simulink model "Test_Encoder_4_to_2"  (Simulink 8.1)
settings: Solver=ode45  StartTime=0.0  StopTime=len  RelTol=1e-3
libraries: commutil2 x2, Encoders_Lib x1
settings Model: Creator=N  LastModifiedBy=uzivatel
settings DataIOCC: LimitDataPoints=off  SignalLoggingSaveFormat=Dataset
settings OptimizationCC: ExpressionDepthLimit=128
settings DebuggingCC: UnderspecifiedInitializationDetection=Simplified  MergeDetectMultiDrivingBlocksExec=error  SolverPrmCheckMsg=none  FcnCallInpInsideContextMsg=EnableAllAsError  FrameProcessingCompatibilityMsg=error  StateNameClashWarn=none
settings HardwareCC: ProdBitPerPointer=64  ProdLargestAtomicFloat=Float  ProdIntDivRoundTo=Zero  ProdEndianess=LittleEndian  ProdHWDeviceType=Intel->x86-64 (Windows64)
settings ModelReferenceCC: PropagateSignalLabelsOutOfModel=on
settings GRTTargetCC: CodeReplacementLibrary=None  CombineOutputUpdateFcns=on  CPPClassGenCompliant=on  GRTInterface=off

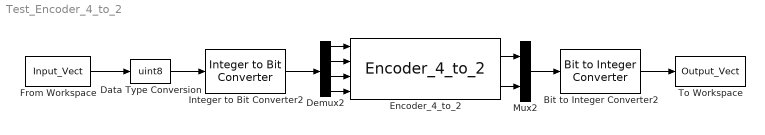
== system Test_Encoder_4_to_2 ==
  Bit to Integer Converter2 : commutil2/Bit to Integer Converter  nbits=2  bitOrder=MSB first  signedOutputValues=Unsigned  outDtype=uint8  outDtypeSigned=Inherit via internal rule
  Data Type Conversion : DataTypeConversion  OutDataTypeStr=uint8
  Demux2 : Demux
  Encoder_4_to_2 : Encoders_Lib/Encoders_Lib/Encoder_4_to_2
  From Workspace : FromWorkspace  VariableName=Input_Vect  SampleTime=1  Interpolate=off  OutputAfterFinalValue=Holding final value
  Integer to Bit Converter2 : commutil2/Integer to Bit Converter  nbits=4  signedInputValues=Unsigned  bitOrder=MSB first  outDtype=boolean
  Mux2 : Mux  Inputs=2
  To Workspace : ToWorkspace  VariableName=Output_Vect  SampleTime=1
  wires:
  Integer to Bit Converter2/1 -> Demux2/1
  Demux2/4 -> Encoder_4_to_2/4
  Demux2/3 -> Encoder_4_to_2/3
  Demux2/2 -> Encoder_4_to_2/2
  Demux2/1 -> Encoder_4_to_2/1
  Mux2/1 -> Bit to Integer Converter2/1
  Bit to Integer Converter2/1 -> To Workspace/1
  Encoder_4_to_2/1 -> Mux2/1
  Encoder_4_to_2/2 -> Mux2/2
  Data Type Conversion/1 -> Integer to Bit Converter2/1
  From Workspace/1 -> Data Type Conversion/1
